simulink model "test_synctime"  (Simulink 8.3)
settings: Solver=ode3  StartTime=0.0  StopTime=Inf  FixedStep=0.01  RelTol=1e-3
libraries: simulink x1, powerlib_extras x1
settings Model: Creator=skills  LastModifiedBy=eruffaldi
settings OptimizationCC: ExpressionDepthLimit=2147483647  InitFltsAndDblsToZero=on
settings DebuggingCC: SaveWithParameterizedLinksMsg=none  SignalResolutionControl=TryResolveAllWithWarning  FcnCallInpInsideContextMsg=UseLocalSettings
settings GRTTargetCC: TargetFcnLib=ansi_tfl_tmw.mat

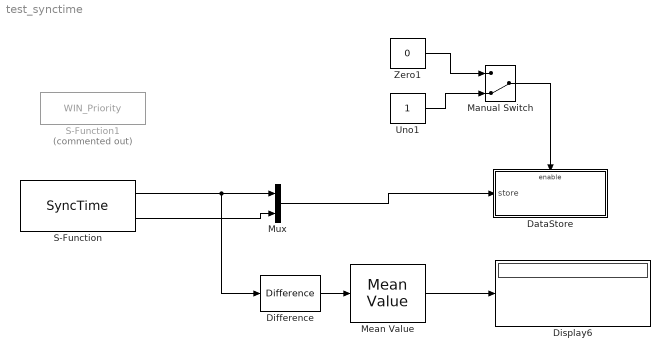
== system test_synctime ==
  DataStore : Subsystem  TreatAsAtomicUnit=on
  Difference : simulink/Discrete/Difference  ICPrevInput=0.0  InputProcessing=Inherited  OutMin=[]  OutMax=[]  OutDataType=fixdt(1, 16)  OutScaling=2^-10  DoSatur=off
  Display6 : Display
  Manual Switch : ManualSwitch  CurrentSetting=0
  Mean Value : powerlib_extras/Measurements/Mean Value  Period=2
  Mux : Mux  Inputs=2
  S-Function : S-Function  Priority=1024  FunctionName=SyncTime  Parameters=dt  EnableBusSupport=off  mask{dt=0.1}
      mask prompts: dt "Period (s) or 0 for sleepless"
      mask Display:
      | port_label('output',1,'Unix Epoch s');
      | port_label('output',2,'Slept s');
  S-Function1 : S-Function  Priority=1024  Commented=on  FunctionName=WIN_Priority  Parameters=pri,thpri,aff  EnableBusSupport=off  mask{pri=1, thpri=1, aff=0}
      mask prompts: pri "Process Priority (+2 +1 0 -1)"; thpri "Thread Priority (+2 +1 0 -1)"; aff "Affinity Mask (bitmask, 0=all)"
  Uno1 : Constant
  Zero1 : Constant  Value=0
  wires:
  Zero1/1 -> Manual Switch/1
  Uno1/1 -> Manual Switch/2
  Manual Switch/1 -> DataStore/Enable
  Mean Value/1 -> Display6/1
  Difference/1 -> Mean Value/1
  S-Function/1 -> Difference/1, Mux/1
  S-Function/2 -> Mux/2
  Mux/1 -> DataStore/1(store)

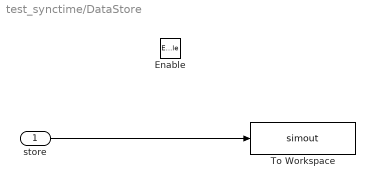
== system test_synctime/DataStore ==
  store : Inport
  Enable : EnablePort
  To Workspace : ToWorkspace  VariableName=simout  SaveFormat=Structure  SampleTime=-1
  wires:
  store/1 -> To Workspace/1
